simulink model "Queue_Model"  (R2023a)
settings: Solver=VariableStepAuto  StartTime=0.0  StopTime=10.0  RelTol=1e-3
libraries: NSA_DEVS_SINKS_ATOMIC x4, NSA_DEVS_SOURCES_ATOMIC x2, NSA_DEVS_LOGISTICS_ATOMIC x2
settings Model: Creator=david  LastModifiedBy=david

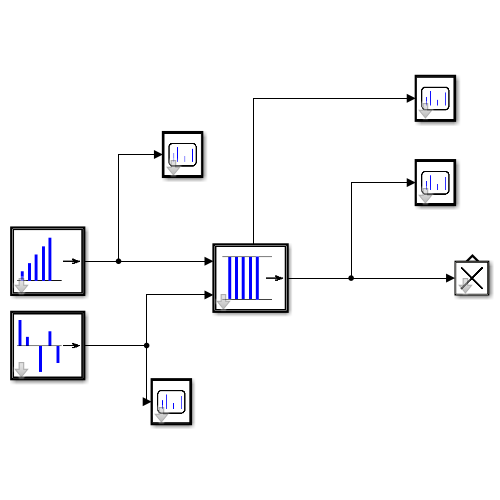
[thumbnail: Simulink's stored preview of the top-level diagram]
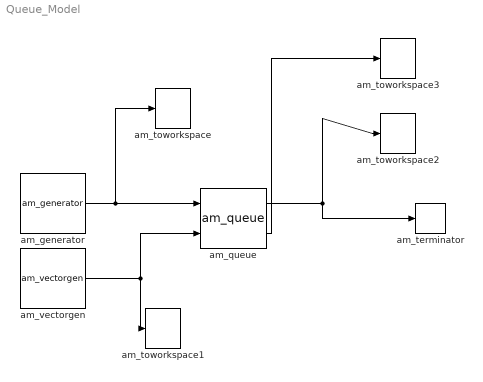
== system Queue_Model ==
  am_generator : NSA_DEVS_SOURCES_ATOMIC/am_generator  tG=1  n0=1  nG=100  tau=[0,1]  debug=0
      settings: SourceProductName=NSA_DEVS
  am_queue : NSA_DEVS_LOGISTICS_ATOMIC/am_queue  tD=[0,2]  tau=[0,1]  debug=0
      settings: SourceProductName=NSA_DEVS
  am_terminator : NSA_DEVS_LOGISTICS_ATOMIC/am_terminator  tau=[0,1]  debug=0
      settings: SourceProductName=NSA_DEVS
  am_toworkspace : NSA_DEVS_SINKS_ATOMIC/am_toworkspace  varname="\"genOut\""  t0=0  format="\"vector\""  tau=[0,1]  debug=0
      settings: SourceProductName=NSA_DEVS
  am_toworkspace1 : NSA_DEVS_SINKS_ATOMIC/am_toworkspace  varname="\"vgenOut\""  t0=0  format="\"vector\""  tau=[0,1]  debug=0
      settings: SourceProductName=NSA_DEVS
  am_toworkspace2 : NSA_DEVS_SINKS_ATOMIC/am_toworkspace  varname="\"queOut\""  t0=0  format="\"vector\""  tau=[0,1]  debug=0
      settings: SourceProductName=NSA_DEVS
  am_toworkspace3 : NSA_DEVS_SINKS_ATOMIC/am_toworkspace  varname="\"queNOut\""  t0=0  format="\"vector\""  tau=[0,1]  debug=0
      settings: SourceProductName=NSA_DEVS
  am_vectorgen : NSA_DEVS_SOURCES_ATOMIC/am_vectorgen  tvec=[0.1 4.5 7.5 9.0 11.0 100]  yvec="[\"1\" \"0\" \"1\" \"0\" \"1\" \"1\"]"  tau=[0,1]  debug=0
      settings: SourceProductName=NSA_DEVS
  wires:
  am_generator/1 -> am_toworkspace/1, am_queue/1
  am_queue/1 -> am_toworkspace2/1, am_terminator/1
  am_vectorgen/1 -> am_toworkspace1/1, am_queue/2
  am_queue/2 -> am_toworkspace3/1
